simulink model "PD_test"  (R2018b)
settings: Solver=VariableStepAuto  StartTime=0.0  StopTime=10.0  RelTol=1e-3
undefined symbols (not defined in the file or in its folder): a_1, a_2
libraries: simulink x2
settings Model: Creator=first  LastModifiedBy=first

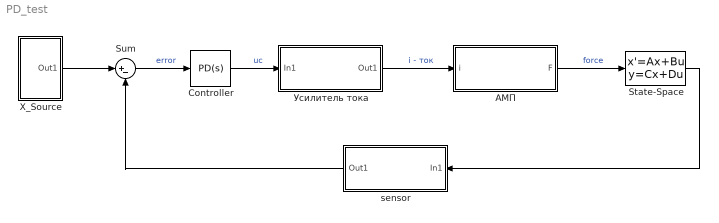
== system PD_test ==
  " Controller" : simulink/Continuous/PID Controller  Controller=PD  Form=Parallel  TimeDomain=Continuous-time  SampleTime=-1  IntegratorMethod=Forward Euler  FilterMethod=Forward Euler  ControllerParametersSource=internal  P=5e3  I=1  D=6.32  UseFilter=on  N=100  TunerSelectOption=Transfer Function Based (PID Tuner App)  InitialConditionSource=internal  InitialConditionForIntegrator=0  InitialConditionForFilter=0  DifferentiatorICPrevScaledInput=0  ExternalReset=none  TrackingMode=off  Kt=1  LimitOutput=off  UpperSaturationLimit=inf  LowerSaturationLimit=-inf  LinearizeAsGain=on  AntiWindupMode=none  Kb=1  POutMin=[]  POutMax=[]  IOutMin=[]  IOutMax=[]  DOutMin=[]  DOutMax=[]  NOutMin=[]  NOutMax=[]  SumOutMin=[]  SumOutMax=[]  SaturationOutMin=[]  SaturationOutMax=[]  PParamMin=[]  PParamMax=[]  IParamMin=[]  IParamMax=[]  DParamMin=[]  DParamMax=[]  NParamMin=[]  NParamMax=[]  KbParamMin=[]  KbParamMax=[]  KtParamMin=[]  KtParamMax=[]  KbOutMin=[]  KbOutMax=[]  KtOutMin=[]  KtOutMax=[]  IntegratorOutMin=[]  IntegratorOutMax=[]  FilterOutMin=[]  FilterOutMax=[]  SumI1OutMin=[]  SumI1OutMax=[]  SumI2OutMin=[]  SumI2OutMax=[]  SumI3OutMin=[]  SumI3OutMax=[]  SumI4OutMin=[]  SumI4OutMax=[]  SumDOutMin=[]  SumDOutMax=[]  DifferentiatorOutMin=[]  DifferentiatorOutMax=[]  FilterDiffOutCoefMin=[]  FilterDiffOutCoefMax=[]  ReciprocalOutMin=[]  ReciprocalOutMax=[]  SumDenOutMin=[]  SumDenOutMax=[]  SumNumOutMin=[]  SumNumOutMax=[]  DivideOutMin=[]  DivideOutMax=[]  IntegratorContinuousStateAttributes=''  IntegratorStateMustResolveToSignalObject=off  IntegratorRTWStateStorageClass=Auto  FilterContinuousStateAttributes=''  FilterStateMustResolveToSignalObject=off  FilterRTWStateStorageClass=Auto  ParallelPVariant=InternalParameters  IdealPVariant=Disabled  IVariant=Disabled  DVariant=InternalParameters  IntegratorVariant=Disabled  SatVariant=Disabled  AWVariant=Disabled  PCopyVariant=Disabled  TRVariant=Disabled  FdbkBlocksVariant=Forward  IdealPFdbkVariant=Disabled  SatFdbkVariant=Disabled  DerivativeFilterVariant=ContFilter  NVariant=InternalParameters  NCopyVariant=Disabled  FilterICVariant=InternalICsFilter  IntegratorICVariant=Disabled  ExternalResetVariant=Disabled  TRSumVariant=Passthrough  SumFdbkVariant=Disabled  SumVariant=Sum_PD
  State-Space : StateSpace  InitialCondition=0
  Sum : Sum  Inputs=|+-
  X_Source : Subsystem
  sensor : Subsystem
  АМП : Subsystem
  "Усилитель тока " : Subsystem
  wires:
  X_Source/1(Out1) -> Sum/1
  Sum/1 -> " Controller"/1  "error"
  " Controller"/1 -> "Усилитель тока "/1(In1)  "uc"
  "Усилитель тока "/1(Out1) -> АМП/1(i)  "i - ток"
  АМП/1(F) -> State-Space/1  "force"
  State-Space/1 -> sensor/1(In1)
  sensor/1(Out1) -> Sum/2

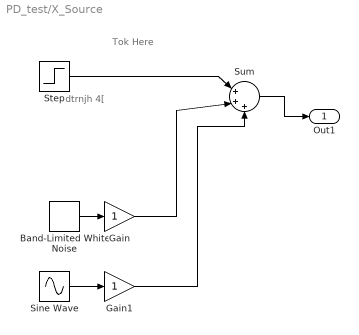
== system PD_test/X_Source ==
  note: Tok Here
  note: dtrnjh 4[
  Band-Limited White Noise : simulink/Sources/Band-Limited White Noise  Cov=[0.1]  Ts=0.1  seed=[23341]
  Gain : Gain
  Gain1 : Gain
  Sine Wave : Sin  SampleTime=0
  Step : Step  SampleTime=0
  Sum : Sum  Inputs=|+++
  Out1 : Outport
  wires:
  Gain1/1 -> Sum/3
  Band-Limited White Noise/1 -> Gain/1
  Sine Wave/1 -> Gain1/1
  Step/1 -> Sum/1
  Gain/1 -> Sum/2
  Sum/1 -> Out1/1

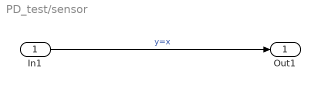
== system PD_test/sensor ==
  In1 : Inport
  Out1 : Outport
  wires:
  In1/1 -> Out1/1  "y=x"

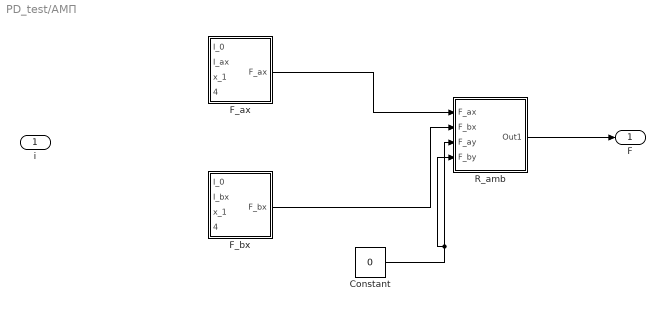
== system PD_test/АМП ==
  i : Inport
  Constant : Constant  Value=0
  F_ax : Subsystem
  F_bx : Subsystem
  R_amb : Subsystem
  F : Outport
  wires:
  F_ax/1(F_ax) -> R_amb/1(F_ax)
  F_bx/1(F_bx) -> R_amb/2(F_bx)
  Constant/1 -> R_amb/4(F_by), R_amb/3(F_ay)
  R_amb/1(Out1) -> F/1

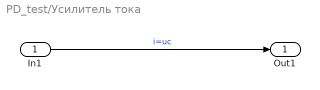
== system PD_test/Усилитель тока  ==
  In1 : Inport
  Out1 : Outport
  wires:
  In1/1 -> Out1/1  "i=uc"

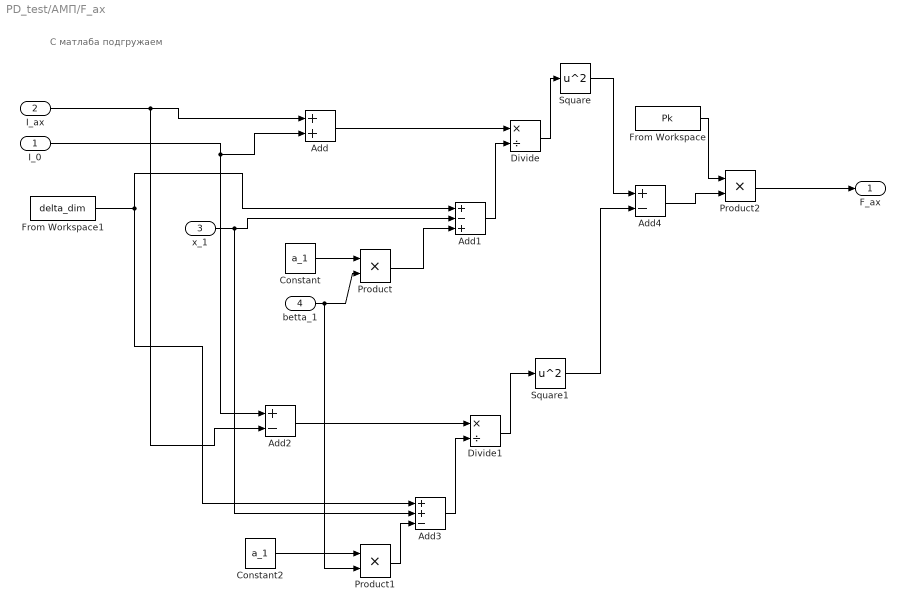
== system PD_test/АМП/F_ax ==
  note: С матлаба подгружаем
  I_0 : Inport
  I_ax : Inport  Port=2
  x_1 : Inport  Port=3
  betta_1 : Inport  Port=4
  Add : Sum
  Add1 : Sum  Inputs=+-+
  Add2 : Sum  Inputs=+-
  Add3 : Sum  Inputs=++-
  Add4 : Sum  Inputs=+-
  Constant : Constant  Value=a_1
  Constant2 : Constant  Value=a_1
  Divide : Product  Inputs=*/
  Divide1 : Product  Inputs=*/
  From Workspace : FromWorkspace  VariableName=Pk  SampleTime=0
  From Workspace1 : FromWorkspace  VariableName=delta_dim  SampleTime=0
  Product : Product
  Product1 : Product
  Product2 : Product
  Square : Math  Operator=square  SaturateOnIntegerOverflow=on
  Square1 : Math  Operator=square  SaturateOnIntegerOverflow=on
  F_ax : Outport
  wires:
  Product2/1 -> F_ax/1
  Constant/1 -> Product/1
  Product/1 -> Add1/3
  Add1/1 -> Divide/2
  Add/1 -> Divide/1
  Divide/1 -> Square/1
  Product1/1 -> Add3/3
  Add2/1 -> Divide1/1
  Constant2/1 -> Product1/1
  I_ax/1 -> Add2/2, Add/1
  Add3/1 -> Divide1/2
  x_1/1 -> Add1/2, Add3/2
  From Workspace1/1 -> Add1/1, Add3/1
  Divide1/1 -> Square1/1
  I_0/1 -> Add/2, Add2/1
  betta_1/1 -> Product/2, Product1/2
  Square/1 -> Add4/1
  Square1/1 -> Add4/2
  From Workspace/1 -> Product2/1
  Add4/1 -> Product2/2

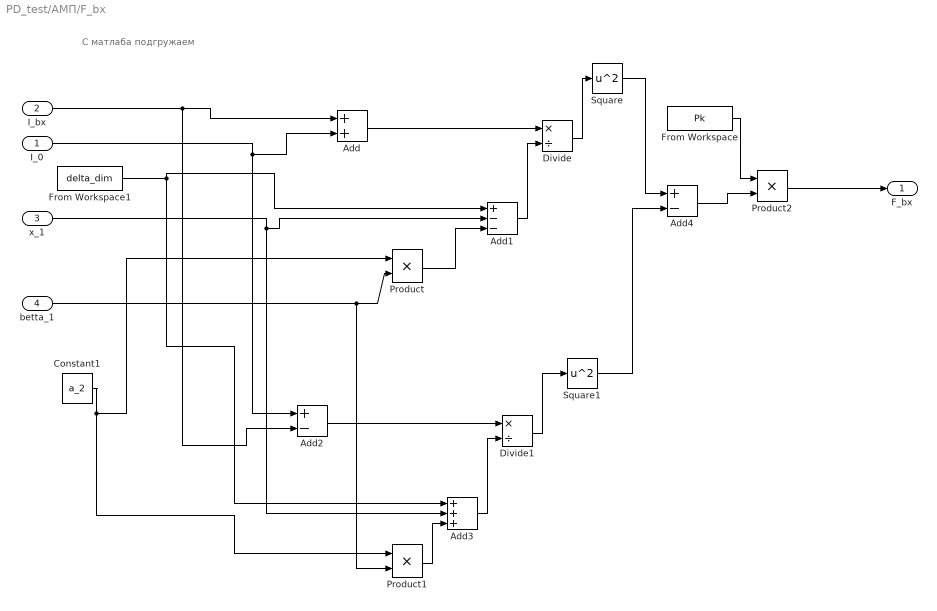
== system PD_test/АМП/F_bx ==
  note: С матлаба подгружаем
  I_0 : Inport
  I_bx : Inport  Port=2
  x_1 : Inport  Port=3
  betta_1 : Inport  Port=4
  Add : Sum
  Add1 : Sum  Inputs=+--
  Add2 : Sum  Inputs=+-
  Add3 : Sum  Inputs=+++
  Add4 : Sum  Inputs=+-
  Constant1 : Constant  Value=a_2
  Divide : Product  Inputs=*/
  Divide1 : Product  Inputs=*/
  From Workspace : FromWorkspace  VariableName=Pk  SampleTime=0
  From Workspace1 : FromWorkspace  VariableName=delta_dim  SampleTime=0
  Product : Product
  Product1 : Product
  Product2 : Product
  Square : Math  Operator=square  SaturateOnIntegerOverflow=on
  Square1 : Math  Operator=square  SaturateOnIntegerOverflow=on
  F_bx : Outport
  wires:
  Product2/1 -> F_bx/1
  Product/1 -> Add1/3
  Add1/1 -> Divide/2
  Add/1 -> Divide/1
  Divide/1 -> Square/1
  Product1/1 -> Add3/3
  Add2/1 -> Divide1/1
  Constant1/1 -> Product1/1, Product/1
  I_bx/1 -> Add2/2, Add/1
  Add3/1 -> Divide1/2
  x_1/1 -> Add1/2, Add3/2
  From Workspace1/1 -> Add1/1, Add3/1
  Divide1/1 -> Square1/1
  I_0/1 -> Add/2, Add2/1
  betta_1/1 -> Product/2, Product1/2
  Square/1 -> Add4/1
  Square1/1 -> Add4/2
  From Workspace/1 -> Product2/1
  Add4/1 -> Product2/2

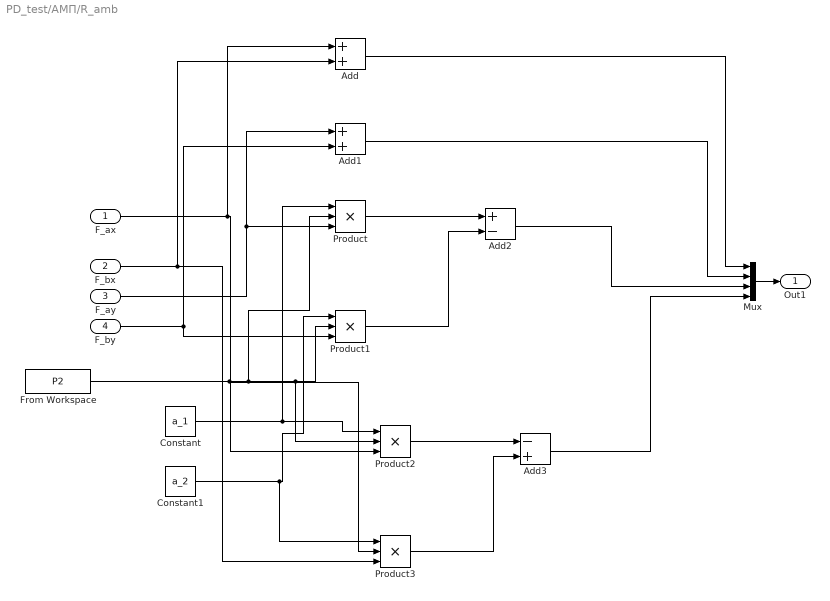
== system PD_test/АМП/R_amb ==
  F_ax : Inport
  F_bx : Inport  Port=2
  F_ay : Inport  Port=3
  F_by : Inport  Port=4
  Add : Sum
  Add1 : Sum
  Add2 : Sum  Inputs=+-
  Add3 : Sum  Inputs=-+
  Constant : Constant  Value=a_1
  Constant1 : Constant  Value=a_2
  From Workspace : FromWorkspace  VariableName=P2  SampleTime=0
  Mux : Mux
  Product{,1..3} (4 alike) : Product  Inputs=3
  Out1 : Outport
  wires:
  F_ax/1 -> Product2/3, Add/1
  F_bx/1 -> Product3/3, Add/2
  Add/1 -> Mux/1
  F_ay/1 -> Product/3, Add1/1
  F_by/1 -> Product1/3, Add1/2
  Add1/1 -> Mux/2
  Mux/1 -> Out1/1
  Constant/1 -> Product2/1, Product/1
  From Workspace/1 -> Product3/2, Product2/2, Product1/2, Product/2
  Product/1 -> Add2/1
  Constant1/1 -> Product3/1, Product1/1
  Product1/1 -> Add2/2
  Add2/1 -> Mux/3
  Product3/1 -> Add3/2
  Product2/1 -> Add3/1
  Add3/1 -> Mux/4
